simulink model "ScenarioManager"  (R2013b)
settings: Solver=ode45  StartTime=0.0  StopTime=10.0  RelTol=1e-3
settings Model: Creator=IT22-ZWPC-208  LastModifiedBy=IT22-ZWPC-208

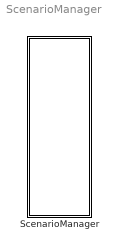
== system ScenarioManager ==
  ScenarioManager : Stateflow chart  TreatAsAtomicUnit=on

== stateflow chart ScenarioManager/ScenarioManager ==
  state AutomaticAction
    state Default
      state LANE_FOLLOW
      state PULL_OVER
      (default) -> LANE_FOLLOW
      LANE_FOLLOW -> PULL_OVER : [SelectPullOverScenario()]
      PULL_OVER -> LANE_FOLLOW
    state Intersection
      state BARE_INTERSECTION_UNPROTECTED
      state STOP_SIGN_PROTECTED
      state STOP_SIGN_UNPROTECTED
      state TRAFFIC_LIGHT_PROTECTED
      state TRAFFIC_LIGHT_UNPROTECTED_LEFT_TURN
      state TRAFFIC_LIGHT_UNPROTECTED_RIGHT_TURN
      state YIELD_SIGN
      (default) -> (junction 71)
      (junction 71) -> BARE_INTERSECTION_UNPROTECTED [order 1] : [SelectBareIntersectionScenario()]
      (junction 71) -> (junction 73) [order 2]
      (junction 73) -> STOP_SIGN_PROTECTED [order 1] : [SelectStopSignScenario()]
      (junction 73) -> (junction 76) [order 2]
      (junction 77) -> TRAFFIC_LIGHT_PROTECTED [order 1]
      (junction 76) -> (junction 77) [order 1] : [SelectTrafficLightScenario()]
      (junction 77) -> TRAFFIC_LIGHT_UNPROTECTED_LEFT_TURN [order 2]
      (junction 77) -> TRAFFIC_LIGHT_UNPROTECTED_RIGHT_TURN [order 3]
      (junction 76) -> (junction 83) [order 2]
      (junction 83) -> YIELD_SIGN : [SelectYieldSignScenario()]
    state PARK_AND_GO
    state Parking
      state VALET_PARKING
      (default) -> VALET_PARKING
    state NARROW_STREET_U_TURN
    state DeadEnd
      state DEADEND_TURNAROUND
      (default) -> DEADEND_TURNAROUND
    state LEARNING_MODEL_SAMPLE
    (default) -> Default
    Default -> PARK_AND_GO [order 1] : SelectParkAndGoScenario()
    PARK_AND_GO -> (junction 52) : [GetStatus()]
    (junction 52) -> Default
    Default -> (junction 67) [order 2]
    (junction 67) -> Intersection [order 1] : [SelectInterceptionScenario()]
    (junction 58) -> (junction 52)
    (junction 67) -> (junction 88) [order 2]
    Parking -> (junction 58) : [GetStatus()]
    (junction 54) -> (junction 58)
    (junction 88) -> Parking [order 1] : [SelectValetParkingScenario()]
    (junction 88) -> (junction 93) [order 2]
    DeadEnd -> (junction 54) : [JudgeReachTargetPoint()]
    (junction 93) -> DeadEnd : [SelectDeadEndScenario()]
    (junction 62) -> (junction 54)
    Intersection -> (junction 62) : [GetStatus()]
  state DriverAction
    state EMERGENCY_STOP
    state EMERGENCY_PULL_OVER
  (default) -> AutomaticAction
  DriverAction -> PARK_AND_GO : [SelectPadMsgScenario()::DrivingAction::RESUME_CRUISE]
  AutomaticAction -> EMERGENCY_STOP [order 1] : [SelectPadMsgScenario()::DrivingAction::STOP]
  AutomaticAction -> EMERGENCY_PULL_OVER [order 2] : [SelectPadMsgScenario()::DrivingAction::PULL_OVER]
